simulink library "SG_library"  (R2020a)
settings: Solver=VariableStepAuto  StartTime=0.0  StopTime=10.0  RelTol=1e-3
undefined symbols (not defined in the file): a, b, c, IO334, IO397
libraries: speedgoatlib_hdlCoder_IO3xx x54, $bdroot x8, hdlsllib x7, simulink x1, simulink_extras x1
(part 1 of 2)
settings Model: Creator=mavolery  LastModifiedBy=padlewsk
settings SFSimCC: CustomCodeUndefinedFunction=UseInterfaceOnly

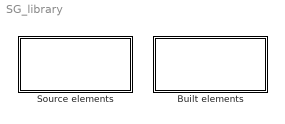
== system SG_library ==
  Built elements : Subsystem
  Source elements : Subsystem

== system SG_library/Built elements ==
  IO334_IO : Subsystem  mask(IO334 IO){}
      mask help: Links the four first physical analog inputs/outputs to the CPU part of the speedgoat.
  IO334_SOS : Subsystem  mask(IO334 M){}
      mask help: Implements a discrete fixed-point filter by second order sections cascade. SOS matrices are given by tf2sos or zp2sos.
  IO397_IO : Subsystem  mask(IO334 IO){}
      mask help: Links the four first physical analog inputs/outputs to the CPU part of the speedgoat.
  IO397_SOS : Subsystem  mask(IO334 IO){}
      mask help: Links the four first physical analog inputs/outputs to the CPU part of the speedgoat.

== system SG_library/Source elements ==
  ADC trigger : Subsystem  mask(AI trigger){}
      mask help: Creates a boolean pulse every given cylces. It can be use for ADC acquisition
  ADC trigger held : Subsystem  mask(AI trigger held){nHeld=2}
      mask prompts: nHeld "Cycles held"
      mask help: Creates a boolean pulse on 'trig' every given cylces. It can be use for ADC acquisition. On 'trig_held' the signal is held to have a for a given number of cycles.
  Discrete SOS section FXP : Subsystem  mask(Discrete fixed-point SOS section){idx=1}
      mask prompts: idx "Index"
      mask help:
      | This is a fixed-point implementation of a biquad filter. Specify the sos [N/2, 6] matrix e.g. given by tf2sos or zpk2sos functions. The first denominator coefficient must always be equal to 1. Index (1 - N/2) parameter specifies which section of the filter is implemented.
      |
      | This is the same implementation as in LabView VI "Discrete Transfer Function Direct.vi" or order 2. It has same fixed-point implementation too.
  Discrete SOS FXP : Subsystem  mask(Discrete fixed-point second order sections filter){sigDataType=fixdt(1,32,16), coefDataType=fixdt(1,32,20)}
      mask prompts: sigDataType "Signal data type"; coefDataType "Coef. data type"
      mask help: This is a SOS implemetation of order 8 (4 sections). Specify the sos [n/2, 6] matrix e.g. given by tf2sos function. The first denominator coefficient must always be equal to 1.
      mask DialogControl Container2 Prompt: Parameters
  Get ADC ticks : Subsystem  mask(Get ADC ticks){}
      mask help: Returns the nuber of FPGA cycles between two ADC acquisitions, given the FPGA clock freuency, the FPGA oversampling factor and the desired acquisition rate.
  Random source : Subsystem  mask(Random source){mean=0, stdev=1, seed=0, SampleTime=0.0001}
      mask prompts: stdev "Standard deviation"; SampleTime "Sample time"
      mask help: Creates some random signal, limited in frequency at Fs/4
  Resettable unit delay : Subsystem  mask(Resettable unit delay){}
      mask Display: dpoly([0 1],[1 0],'z');
  Triggered Pulse : Subsystem  mask(Triggered Pulse){}
      mask help: Generates a single pulse of N samples length

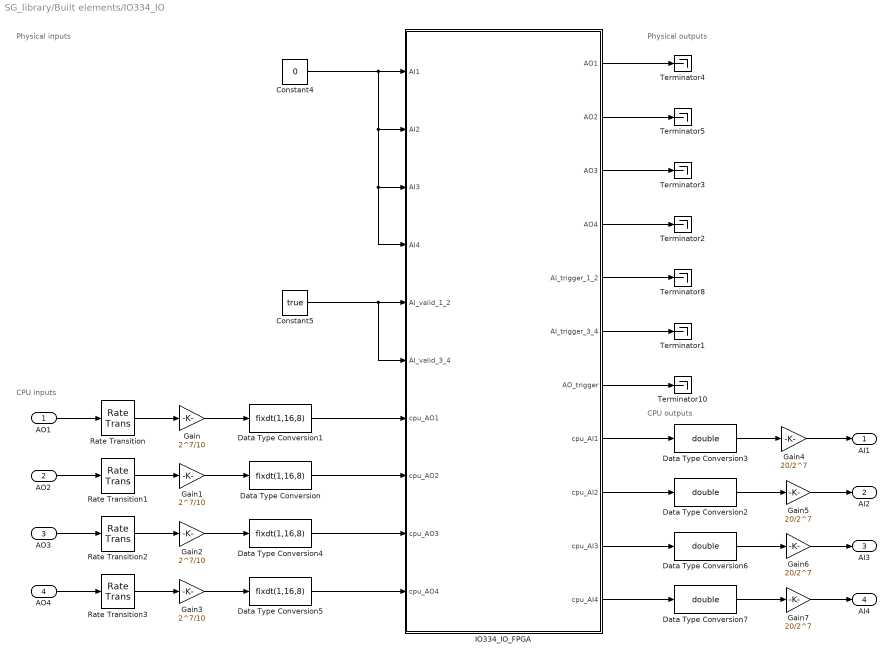
== system SG_library/Built elements/IO334_IO ==
  note: CPU outputs
  note: Physical outputs
  note: Physical inputs
  note: CPU inputs
  AO1 : Inport
  AO2 : Inport  Port=2
  AO3 : Inport  Port=3
  AO4 : Inport  Port=4
  Constant4 : Constant  Value=0  OutDataTypeStr=fixdt(1,16,8)  SampleTime=-1
  Constant5 : Constant  Value=true  SampleTime=-1
  Data Type Conversion{,1,4..5} (4 alike) : DataTypeConversion  OutDataTypeStr=fixdt(1,16,8)
  Data Type Conversion{2..3,6..7} (4 alike) : DataTypeConversion  OutDataTypeStr=double
  Gain{,1..3} (4 alike) : Gain  Gain=2^7/10
  Gain{4..7} (4 alike) : Gain  Gain=20/2^7
  IO334_IO_FPGA : Subsystem  mask(Speedgoat IO334-325k Interface Block){module_id=1, slot=-1, ts=-1, OutputRange=Auto (same as ADC), FpgaFreq=100}
      mask prompts: module_id "FPGA Module Identifier:"; slot "PCI slot (-1: autosearch):"; ts "Sample time:"; OutputRange "DAC Voltage Range:"; FpgaFreq "FPGA Frequency [MHz]"
      mask help: Simulink Real-Time Interface Block for Speedgoat IO334-325k.
      mask init:
      | mfpgaparameters;
      mask Help: eval('speedgoatdoc_hdlc')
      mask TypeOptions OutputRange: IO334 DAC Setup/OutputRange
      mask DialogControl AnalogOutput Prompt: Analog Output
      mask Display:
      | SetupBlkPath = find_system(gcb, 'LookUnderMasks', 'all', 'FollowLinks', 'on', 'regexp', 'on', 'Name', 'IO3(\d|x){2}\s+Setup' );
      | SetupBlkPath = SetupBlkPath{1};
      | TS = get_param(SetupBlkPath,'timestamp_mcs');
      | disp(sprintf('Speedgoat IO334-325k\nFPGA I/O Module\n\nTimestamp\n%s\n\nReference Design\nVersion 1.2\n\nMatlab R2020a\n\nPCIe Link Width: X4\nRear Plugin: None\nAurora Mode: None\nAurora Byteswap: true\n', TS))
  Rate Transition{,1..3} (4 alike) : RateTransition
  Terminator{1..5,8,10} (7 alike) : Terminator
  AI1 : Outport  VectorParamsAs1DForOutWhenUnconnected=off
  AI2 : Outport  Port=2  VectorParamsAs1DForOutWhenUnconnected=off
  AI3 : Outport  Port=3  VectorParamsAs1DForOutWhenUnconnected=off
  AI4 : Outport  Port=4  VectorParamsAs1DForOutWhenUnconnected=off
  wires:
  AO1/1 -> Rate Transition/1
  AO2/1 -> Rate Transition1/1
  Rate Transition/1 -> Gain/1
  Rate Transition1/1 -> Gain1/1
  Data Type Conversion3/1 -> Gain4/1
  Data Type Conversion2/1 -> Gain5/1
  Rate Transition2/1 -> Gain2/1
  AO3/1 -> Rate Transition2/1
  Rate Transition3/1 -> Gain3/1
  AO4/1 -> Rate Transition3/1
  Data Type Conversion5/1 -> IO334_IO_FPGA/10(cpu_AO4)
  Data Type Conversion/1 -> IO334_IO_FPGA/8(cpu_AO2)
  Data Type Conversion4/1 -> IO334_IO_FPGA/9(cpu_AO3)
  Data Type Conversion1/1 -> IO334_IO_FPGA/7(cpu_AO1)
  Data Type Conversion6/1 -> Gain6/1
  Data Type Conversion7/1 -> Gain7/1
  IO334_IO_FPGA/1(AO1) -> Terminator4/1
  IO334_IO_FPGA/8(cpu_AI1) -> Data Type Conversion3/1
  IO334_IO_FPGA/9(cpu_AI2) -> Data Type Conversion2/1
  IO334_IO_FPGA/10(cpu_AI3) -> Data Type Conversion6/1
  IO334_IO_FPGA/11(cpu_AI4) -> Data Type Conversion7/1
  IO334_IO_FPGA/7(AO_trigger) -> Terminator10/1
  IO334_IO_FPGA/6(AI_trigger_3_4) -> Terminator1/1
  IO334_IO_FPGA/5(AI_trigger_1_2) -> Terminator8/1
  IO334_IO_FPGA/4(AO4) -> Terminator2/1
  IO334_IO_FPGA/3(AO3) -> Terminator3/1
  IO334_IO_FPGA/2(AO2) -> Terminator5/1
  Gain/1 -> Data Type Conversion1/1
  Gain1/1 -> Data Type Conversion/1
  Gain2/1 -> Data Type Conversion4/1
  Gain3/1 -> Data Type Conversion5/1
  Gain4/1 -> AI1/1
  Gain5/1 -> AI2/1
  Gain6/1 -> AI3/1
  Gain7/1 -> AI4/1
  Constant5/1 -> IO334_IO_FPGA/6(AI_valid_3_4), IO334_IO_FPGA/5(AI_valid_1_2)
  Constant4/1 -> IO334_IO_FPGA/2(AI2), IO334_IO_FPGA/3(AI3), IO334_IO_FPGA/4(AI4), IO334_IO_FPGA/1(AI1)

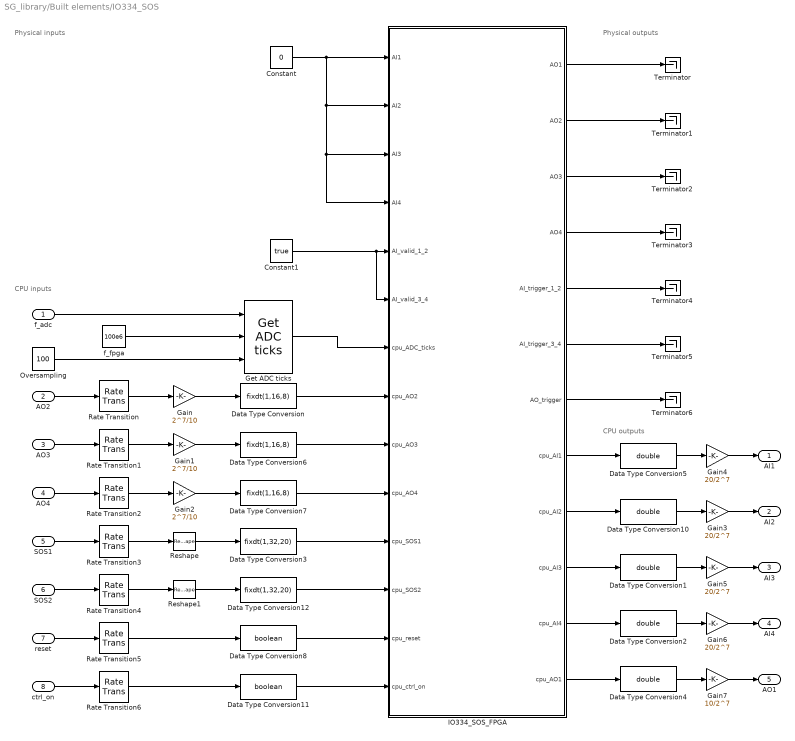
== system SG_library/Built elements/IO334_SOS ==
  note: Physical inputs
  note: CPU inputs
  note: CPU outputs
  note: Physical outputs
  f_adc : Inport
  AO2 : Inport  Port=2
  AO3 : Inport  Port=3
  AO4 : Inport  Port=4
  SOS1 : Inport  Port=5
  SOS2 : Inport  Port=6
  reset : Inport  Port=7
  ctrl_on : Inport  Port=8
  Constant : Constant  Value=0  OutDataTypeStr=fixdt(1,16,8)  SampleTime=-1
  Constant1 : Constant  Value=true  SampleTime=-1
  Data Type Conversion : DataTypeConversion  OutDataTypeStr=fixdt(1,16,8)
  Data Type Conversion{1..2,4..5,10} (5 alike) : DataTypeConversion  OutDataTypeStr=double
  Data Type Conversion11 : DataTypeConversion  OutDataTypeStr=boolean
  Data Type Conversion12 : DataTypeConversion  OutDataTypeStr=fixdt(1,32,20)
  Data Type Conversion3 : DataTypeConversion  OutDataTypeStr=fixdt(1,32,20)
  Data Type Conversion6 : DataTypeConversion  OutDataTypeStr=fixdt(1,16,8)
  Data Type Conversion7 : DataTypeConversion  OutDataTypeStr=fixdt(1,16,8)
  Data Type Conversion8 : DataTypeConversion  OutDataTypeStr=boolean
  Gain : Gain  Gain=2^7/10
  Gain1 : Gain  Gain=2^7/10
  Gain2 : Gain  Gain=2^7/10
  Gain{3..6} (4 alike) : Gain  Gain=20/2^7
  Gain7 : Gain  Gain=10/2^7
  Get ADC ticks : $bdroot/Source elements/Get ADC ticks
  IO334_SOS_FPGA : Subsystem  mask(Speedgoat IO334-325k Interface Block){module_id=1, slot=-1, ts=-1, OutputRange=Auto (same as ADC), FpgaFreq=100}
      mask prompts: module_id "FPGA Module Identifier:"; slot "PCI slot (-1: autosearch):"; ts "Sample time:"; OutputRange "DAC Voltage Range:"; FpgaFreq "FPGA Frequency [MHz]"
      mask help: Simulink Real-Time Interface Block for Speedgoat IO334-325k.
      mask init:
      | mfpgaparameters;
      mask Help: eval('speedgoatdoc_hdlc')
      mask TypeOptions OutputRange: IO334 DAC Setup/OutputRange
      mask DialogControl AnalogOutput Prompt: Analog Output
      mask Display:
      | SetupBlkPath = find_system(gcb, 'LookUnderMasks', 'all', 'FollowLinks', 'on', 'regexp', 'on', 'Name', 'IO3(\d|x){2}\s+Setup' );
      | SetupBlkPath = SetupBlkPath{1};
      | TS = get_param(SetupBlkPath,'timestamp_mcs');
      | disp(sprintf('Speedgoat IO334-325k\nFPGA I/O Module\n\nTimestamp\n%s\n\nReference Design\nVersion 1.2\n\nMatlab R2020a\n\nPCIe Link Width: X4\nRear Plugin: None\nAurora Mode: None\nAurora Byteswap: true\n', TS))
  Oversampling : Constant  Value=100  SampleTime=-1
  Rate Transition{,1..6} (7 alike) : RateTransition
  Reshape : Reshape
  Reshape1 : Reshape
  Terminator{,1..6} (7 alike) : Terminator
  f_fpga : Constant  Value=100e6  SampleTime=-1
  AI1 : Outport  VectorParamsAs1DForOutWhenUnconnected=off
  AI2 : Outport  Port=2  VectorParamsAs1DForOutWhenUnconnected=off
  AI3 : Outport  Port=3  VectorParamsAs1DForOutWhenUnconnected=off
  AI4 : Outport  Port=4  VectorParamsAs1DForOutWhenUnconnected=off
  AO1 : Outport  Port=5  VectorParamsAs1DForOutWhenUnconnected=off
  wires:
  Data Type Conversion10/1 -> Gain3/1
  Data Type Conversion5/1 -> Gain4/1
  Data Type Conversion1/1 -> Gain5/1
  Data Type Conversion2/1 -> Gain6/1
  IO334_SOS_FPGA/1(AO1) -> Terminator/1
  IO334_SOS_FPGA/2(AO2) -> Terminator1/1
  IO334_SOS_FPGA/3(AO3) -> Terminator2/1
  IO334_SOS_FPGA/4(AO4) -> Terminator3/1
  IO334_SOS_FPGA/5(AI_trigger_1_2) -> Terminator4/1
  IO334_SOS_FPGA/6(AI_trigger_3_4) -> Terminator5/1
  IO334_SOS_FPGA/7(AO_trigger) -> Terminator6/1
  IO334_SOS_FPGA/8(cpu_AI1) -> Data Type Conversion5/1
  IO334_SOS_FPGA/9(cpu_AI2) -> Data Type Conversion10/1
  IO334_SOS_FPGA/10(cpu_AI3) -> Data Type Conversion1/1
  IO334_SOS_FPGA/11(cpu_AI4) -> Data Type Conversion2/1
  Rate Transition3/1 -> Reshape/1
  Rate Transition/1 -> Gain/1
  Rate Transition1/1 -> Gain1/1
  Rate Transition2/1 -> Gain2/1
  AO2/1 -> Rate Transition/1
  AO3/1 -> Rate Transition1/1
  AO4/1 -> Rate Transition2/1
  Rate Transition5/1 -> Data Type Conversion8/1
  reset/1 -> Rate Transition5/1
  Rate Transition6/1 -> Data Type Conversion11/1
  ctrl_on/1 -> Rate Transition6/1
  Data Type Conversion/1 -> IO334_SOS_FPGA/8(cpu_AO2)
  Data Type Conversion6/1 -> IO334_SOS_FPGA/9(cpu_AO3)
  Data Type Conversion7/1 -> IO334_SOS_FPGA/10(cpu_AO4)
  Data Type Conversion11/1 -> IO334_SOS_FPGA/14(cpu_ctrl_on)
  Data Type Conversion8/1 -> IO334_SOS_FPGA/13(cpu_reset)
  Constant1/1 -> IO334_SOS_FPGA/5(AI_valid_1_2), IO334_SOS_FPGA/6(AI_valid_3_4)
  Constant/1 -> IO334_SOS_FPGA/1(AI1), IO334_SOS_FPGA/2(AI2), IO334_SOS_FPGA/3(AI3), IO334_SOS_FPGA/4(AI4)
  SOS1/1 -> Rate Transition3/1
  Data Type Conversion3/1 -> IO334_SOS_FPGA/11(cpu_SOS1)
  f_adc/1 -> Get ADC ticks/1
  Oversampling/1 -> Get ADC ticks/3
  f_fpga/1 -> Get ADC ticks/2
  Data Type Conversion4/1 -> Gain7/1
  IO334_SOS_FPGA/12(cpu_AO1) -> Data Type Conversion4/1
  Rate Transition4/1 -> Reshape1/1
  SOS2/1 -> Rate Transition4/1
  Data Type Conversion12/1 -> IO334_SOS_FPGA/12(cpu_SOS2)
  Gain/1 -> Data Type Conversion/1
  Gain1/1 -> Data Type Conversion6/1
  Gain2/1 -> Data Type Conversion7/1
  Reshape/1 -> Data Type Conversion3/1
  Reshape1/1 -> Data Type Conversion12/1
  Get ADC ticks/1 -> IO334_SOS_FPGA/7(cpu_ADC_ticks)
  Gain4/1 -> AI1/1
  Gain3/1 -> AI2/1
  Gain5/1 -> AI3/1
  Gain6/1 -> AI4/1
  Gain7/1 -> AO1/1

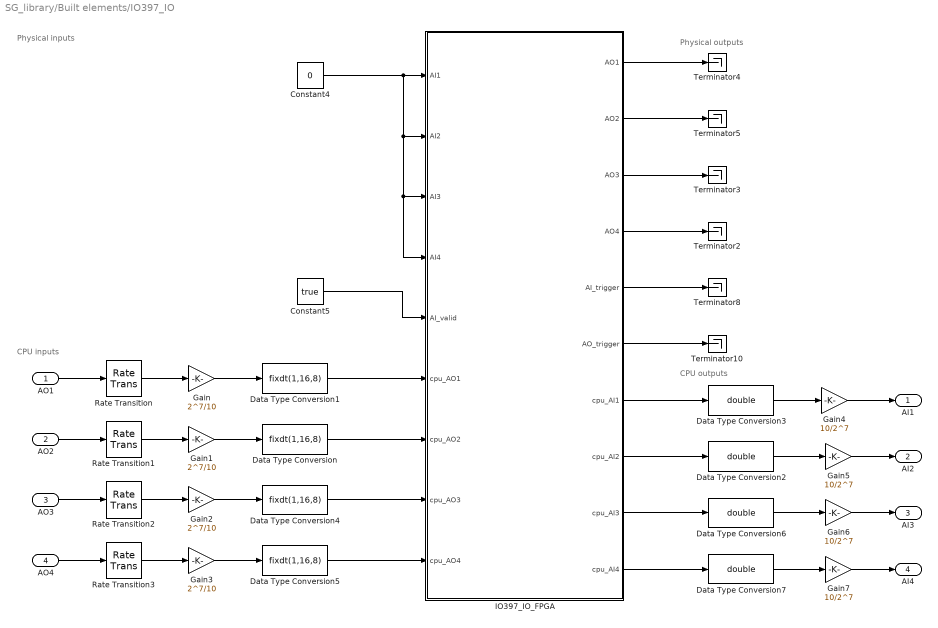
== system SG_library/Built elements/IO397_IO ==
  note: CPU outputs
  note: Physical outputs
  note: Physical inputs
  note: CPU inputs
  AO1 : Inport
  AO2 : Inport  Port=2
  AO3 : Inport  Port=3
  AO4 : Inport  Port=4
  Constant4 : Constant  Value=0  OutDataTypeStr=fixdt(1,16,8)  SampleTime=-1
  Constant5 : Constant  Value=true  SampleTime=-1
  Data Type Conversion{,1,4..5} (4 alike) : DataTypeConversion  OutDataTypeStr=fixdt(1,16,8)  SaturateOnIntegerOverflow=on
  Data Type Conversion{2..3,6..7} (4 alike) : DataTypeConversion  OutDataTypeStr=double
  Gain{,1..3} (4 alike) : Gain  Gain=2^7/10
  Gain{4..7} (4 alike) : Gain  Gain=10/2^7
  IO397_IO_FPGA : Subsystem  mask(Speedgoat IO397-50k Interface Block){module_id=1, slot=-1, ts=-1, range1=+-10 V, range2=+-10 V, range3=+-10 V, range4=+-10 V, span=+-10 V, FpgaFreq=100}
      mask prompts: module_id "FPGA Module Identifier:"; slot "PCI slot (-1: autosearch):"; ts "Sample time:"; range1 "Range ADC Channel 1"; range2 "Range ADC Channel 2"; range3 "Range ADC Channel 3"; range4 "Range ADC Channel 4"; span "DAC Voltage Span:"; FpgaFreq "FPGA Frequency [MHz]"
      mask help: Simulink Real-Time Interface Block for Speedgoat IO397-50k.
      mask init:
      | mfpgaparameters;
      mask Help: eval('speedgoatdoc_hdlc')
      mask TypeOptions range1: IO397 ADC Setup/range1
      mask TypeOptions range2: IO397 ADC Setup/range2
      mask TypeOptions range3: IO397 ADC Setup/range3
      mask TypeOptions range4: IO397 ADC Setup/range4
      mask TypeOptions span: IO397 DAC Setup/span
      mask DialogControl AnalogInput Prompt: Analog Input
      mask DialogControl AnalogOutput Prompt: Analog Output
      mask Display:
      | SetupBlkPath = find_system(gcb, 'LookUnderMasks', 'all', 'FollowLinks', 'on', 'regexp', 'on', 'Name', 'IO3(\d|x){2}\s+Setup' );
      | SetupBlkPath = SetupBlkPath{1};
      | TS = get_param(SetupBlkPath,'timestamp_mcs');
      | disp(sprintf('Speedgoat IO397-50k\nFPGA I/O Module\n\nTimestamp\n%s\n\nReference Design\nVersion 1.2\n\nMatlab R2020a\n\nPCIe Link Width: X1\n', TS))
  Rate Transition{,1..3} (4 alike) : RateTransition
  Terminator{2..5,8,10} (6 alike) : Terminator
  AI1 : Outport  VectorParamsAs1DForOutWhenUnconnected=off
  AI2 : Outport  Port=2  VectorParamsAs1DForOutWhenUnconnected=off
  AI3 : Outport  Port=3  VectorParamsAs1DForOutWhenUnconnected=off
  AI4 : Outport  Port=4  VectorParamsAs1DForOutWhenUnconnected=off
  wires:
  AO1/1 -> Rate Transition/1
  AO2/1 -> Rate Transition1/1
  Rate Transition/1 -> Gain/1
  Rate Transition1/1 -> Gain1/1
  Data Type Conversion3/1 -> Gain4/1
  Data Type Conversion2/1 -> Gain5/1
  Rate Transition2/1 -> Gain2/1
  AO3/1 -> Rate Transition2/1
  Rate Transition3/1 -> Gain3/1
  AO4/1 -> Rate Transition3/1
  Data Type Conversion5/1 -> IO397_IO_FPGA/9(cpu_AO4)
  Data Type Conversion/1 -> IO397_IO_FPGA/7(cpu_AO2)
  Data Type Conversion4/1 -> IO397_IO_FPGA/8(cpu_AO3)
  Data Type Conversion1/1 -> IO397_IO_FPGA/6(cpu_AO1)
  Data Type Conversion6/1 -> Gain6/1
  Data Type Conversion7/1 -> Gain7/1
  IO397_IO_FPGA/1(AO1) -> Terminator4/1
  IO397_IO_FPGA/7(cpu_AI1) -> Data Type Conversion3/1
  IO397_IO_FPGA/8(cpu_AI2) -> Data Type Conversion2/1
  IO397_IO_FPGA/9(cpu_AI3) -> Data Type Conversion6/1
  IO397_IO_FPGA/10(cpu_AI4) -> Data Type Conversion7/1
  IO397_IO_FPGA/6(AO_trigger) -> Terminator10/1
  IO397_IO_FPGA/5(AI_trigger) -> Terminator8/1
  IO397_IO_FPGA/4(AO4) -> Terminator2/1
  IO397_IO_FPGA/3(AO3) -> Terminator3/1
  IO397_IO_FPGA/2(AO2) -> Terminator5/1
  Gain/1 -> Data Type Conversion1/1
  Gain1/1 -> Data Type Conversion/1
  Gain2/1 -> Data Type Conversion4/1
  Gain3/1 -> Data Type Conversion5/1
  Gain4/1 -> AI1/1
  Gain5/1 -> AI2/1
  Gain6/1 -> AI3/1
  Gain7/1 -> AI4/1
  Constant5/1 -> IO397_IO_FPGA/5(AI_valid)
  Constant4/1 -> IO397_IO_FPGA/2(AI2), IO397_IO_FPGA/3(AI3), IO397_IO_FPGA/4(AI4), IO397_IO_FPGA/1(AI1)

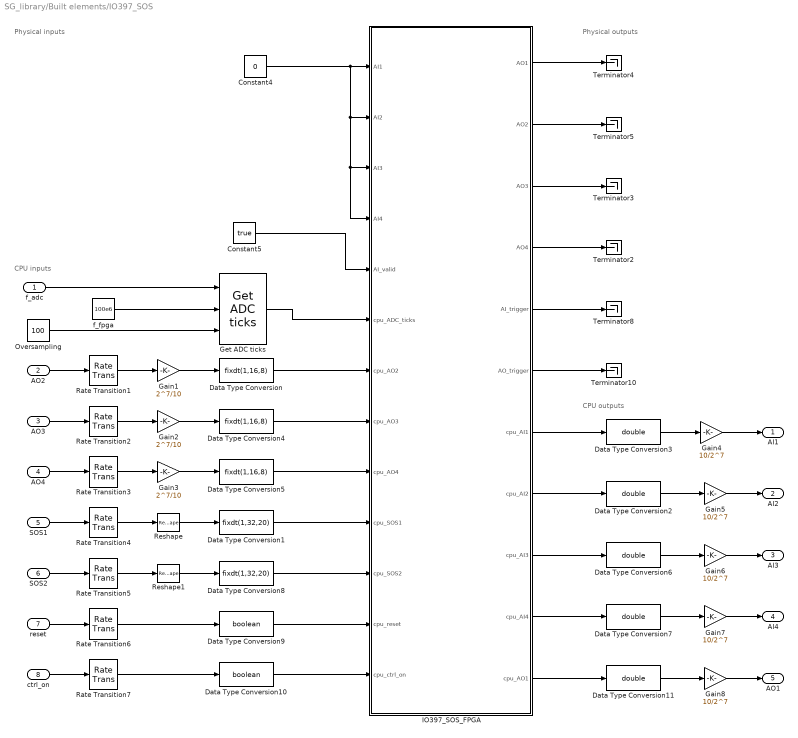
== system SG_library/Built elements/IO397_SOS ==
  note: CPU outputs
  note: Physical outputs
  note: Physical inputs
  note: CPU inputs
  f_adc : Inport
  AO2 : Inport  Port=2
  AO3 : Inport  Port=3
  AO4 : Inport  Port=4
  SOS1 : Inport  Port=5
  SOS2 : Inport  Port=6
  reset : Inport  Port=7
  ctrl_on : Inport  Port=8
  Constant4 : Constant  Value=0  OutDataTypeStr=fixdt(1,16,8)  SampleTime=-1
  Constant5 : Constant  Value=true  SampleTime=-1
  Data Type Conversion : DataTypeConversion  OutDataTypeStr=fixdt(1,16,8)  SaturateOnIntegerOverflow=on
  Data Type Conversion1 : DataTypeConversion  OutDataTypeStr=fixdt(1,32,20)  SaturateOnIntegerOverflow=on
  Data Type Conversion10 : DataTypeConversion  OutDataTypeStr=boolean
  Data Type Conversion{2..3,6..7,11} (5 alike) : DataTypeConversion  OutDataTypeStr=double
  Data Type Conversion4 : DataTypeConversion  OutDataTypeStr=fixdt(1,16,8)  SaturateOnIntegerOverflow=on
  Data Type Conversion5 : DataTypeConversion  OutDataTypeStr=fixdt(1,16,8)  SaturateOnIntegerOverflow=on
  Data Type Conversion8 : DataTypeConversion  OutDataTypeStr=fixdt(1,32,20)  SaturateOnIntegerOverflow=on
  Data Type Conversion9 : DataTypeConversion  OutDataTypeStr=boolean
  Gain1 : Gain  Gain=2^7/10
  Gain2 : Gain  Gain=2^7/10
  Gain3 : Gain  Gain=2^7/10
  Gain{4..8} (5 alike) : Gain  Gain=10/2^7
  Get ADC ticks : $bdroot/Source elements/Get ADC ticks
  IO397_SOS_FPGA : Subsystem  mask(Speedgoat IO397-50k Interface Block){module_id=1, slot=-1, ts=-1, range1=+-10 V, range2=+-10 V, range3=+-10 V, range4=+-10 V, span=+-10 V, FpgaFreq=100}
      mask prompts: module_id "FPGA Module Identifier:"; slot "PCI slot (-1: autosearch):"; ts "Sample time:"; range1 "Range ADC Channel 1"; range2 "Range ADC Channel 2"; range3 "Range ADC Channel 3"; range4 "Range ADC Channel 4"; span "DAC Voltage Span:"; FpgaFreq "FPGA Frequency [MHz]"
      mask help: Simulink Real-Time Interface Block for Speedgoat IO397-50k.
      mask init:
      | mfpgaparameters;
      mask Help: eval('speedgoatdoc_hdlc')
      mask TypeOptions range1: IO397 ADC Setup/range1
      mask TypeOptions range2: IO397 ADC Setup/range2
      mask TypeOptions range3: IO397 ADC Setup/range3
      mask TypeOptions range4: IO397 ADC Setup/range4
      mask TypeOptions span: IO397 DAC Setup/span
      mask DialogControl AnalogInput Prompt: Analog Input
      mask DialogControl AnalogOutput Prompt: Analog Output
      mask Display:
      | SetupBlkPath = find_system(gcb, 'LookUnderMasks', 'all', 'FollowLinks', 'on', 'regexp', 'on', 'Name', 'IO3(\d|x){2}\s+Setup' );
      | SetupBlkPath = SetupBlkPath{1};
      | TS = get_param(SetupBlkPath,'timestamp_mcs');
      | disp(sprintf('Speedgoat IO397-50k\nFPGA I/O Module\n\nTimestamp\n%s\n\nReference Design\nVersion 1.2\n\nMatlab R2020a\n\nPCIe Link Width: X1\n', TS))
  Oversampling : Constant  Value=100
  Rate Transition{1..7} (7 alike) : RateTransition
  Reshape : Reshape
  Reshape1 : Reshape
  Terminator{2..5,8,10} (6 alike) : Terminator
  f_fpga : Constant  Value=100e6
  AI1 : Outport  VectorParamsAs1DForOutWhenUnconnected=off
  AI2 : Outport  Port=2  VectorParamsAs1DForOutWhenUnconnected=off
  AI3 : Outport  Port=3  VectorParamsAs1DForOutWhenUnconnected=off
  AI4 : Outport  Port=4  VectorParamsAs1DForOutWhenUnconnected=off
  AO1 : Outport  Port=5  VectorParamsAs1DForOutWhenUnconnected=off
  wires:
  AO2/1 -> Rate Transition1/1
  Rate Transition1/1 -> Gain1/1
  Data Type Conversion3/1 -> Gain4/1
  Data Type Conversion2/1 -> Gain5/1
  Rate Transition2/1 -> Gain2/1
  AO3/1 -> Rate Transition2/1
  Rate Transition3/1 -> Gain3/1
  AO4/1 -> Rate Transition3/1
  Data Type Conversion5/1 -> IO397_SOS_FPGA/9(cpu_AO4)
  Data Type Conversion/1 -> IO397_SOS_FPGA/7(cpu_AO2)
  Data Type Conversion4/1 -> IO397_SOS_FPGA/8(cpu_AO3)
  Data Type Conversion6/1 -> Gain6/1
  Data Type Conversion7/1 -> Gain7/1
  IO397_SOS_FPGA/1(AO1) -> Terminator4/1
  IO397_SOS_FPGA/7(cpu_AI1) -> Data Type Conversion3/1
  IO397_SOS_FPGA/8(cpu_AI2) -> Data Type Conversion2/1
  IO397_SOS_FPGA/9(cpu_AI3) -> Data Type Conversion6/1
  IO397_SOS_FPGA/10(cpu_AI4) -> Data Type Conversion7/1
  IO397_SOS_FPGA/6(AO_trigger) -> Terminator10/1
  IO397_SOS_FPGA/5(AI_trigger) -> Terminator8/1
  IO397_SOS_FPGA/4(AO4) -> Terminator2/1
  IO397_SOS_FPGA/3(AO3) -> Terminator3/1
  IO397_SOS_FPGA/2(AO2) -> Terminator5/1
  Gain1/1 -> Data Type Conversion/1
  Gain2/1 -> Data Type Conversion4/1
  Gain3/1 -> Data Type Conversion5/1
  Gain4/1 -> AI1/1
  Gain5/1 -> AI2/1
  Gain6/1 -> AI3/1
  Gain7/1 -> AI4/1
  Constant5/1 -> IO397_SOS_FPGA/5(AI_valid)
  Constant4/1 -> IO397_SOS_FPGA/3(AI3), IO397_SOS_FPGA/4(AI4), IO397_SOS_FPGA/2(AI2), IO397_SOS_FPGA/1(AI1)
  ctrl_on/1 -> Rate Transition7/1
  reset/1 -> Rate Transition6/1
  SOS2/1 -> Rate Transition5/1
  SOS1/1 -> Rate Transition4/1
  f_adc/1 -> Get ADC ticks/1
  f_fpga/1 -> Get ADC ticks/2
  Oversampling/1 -> Get ADC ticks/3
  Rate Transition4/1 -> Reshape/1
  Rate Transition5/1 -> Reshape1/1
  Reshape1/1 -> Data Type Conversion8/1
  Reshape/1 -> Data Type Conversion1/1
  Rate Transition6/1 -> Data Type Conversion9/1
  Rate Transition7/1 -> Data Type Conversion10/1
  Data Type Conversion9/1 -> IO397_SOS_FPGA/12(cpu_reset)
  Data Type Conversion10/1 -> IO397_SOS_FPGA/13(cpu_ctrl_on)
  Data Type Conversion8/1 -> IO397_SOS_FPGA/11(cpu_SOS2)
  Data Type Conversion1/1 -> IO397_SOS_FPGA/10(cpu_SOS1)
  Get ADC ticks/1 -> IO397_SOS_FPGA/6(cpu_ADC_ticks)
  Data Type Conversion11/1 -> Gain8/1
  Gain8/1 -> AO1/1
  IO397_SOS_FPGA/11(cpu_AO1) -> Data Type Conversion11/1

== system SG_library/Source elements/ADC trigger ==
  ticks : Inport
  HDL Counter3 : hdlsllib/Sources/HDL Counter  CountType=Free running  CountInit=uint32(0)  CountStep=uint32(1)  CountMax=25  CountFromType=Initial value  CountFrom=uint32(0)  CountResetPort=on  CountLoadPort=off  CountEnbPort=off  CountDirPort=off  CountDataType=Unsigned  CountWordLen=32  CountFracLen=0  CountSampTime=1
  Relational Operator1 : RelationalOperator  Operator=<=  OutDataTypeStr=boolean  RndMeth=Simplest
  trig : Outport  VectorParamsAs1DForOutWhenUnconnected=off
  wires:
  HDL Counter3/1 -> Relational Operator1/2
  ticks/1 -> Relational Operator1/1
  Relational Operator1/1 -> HDL Counter3/1, trig/1

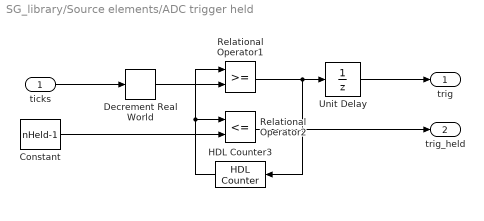
== system SG_library/Source elements/ADC trigger held ==
  ticks : Inport
  Constant : Constant  Value=nHeld-1  OutDataTypeStr=uint32  SampleTime=-1
  Decrement Real World : simulink/Additional Math & Discrete/Additional Math: Increment - Decrement/Decrement Real World
      settings: SourceProductBaseCode=SL
  HDL Counter3 : hdlsllib/Sources/HDL Counter  CountType=Free running  CountInit=uint32(0)  CountStep=uint32(1)  CountMax=25  CountFromType=Initial value  CountFrom=uint32(0)  CountResetPort=on  CountLoadPort=off  CountEnbPort=off  CountDirPort=off  CountDataType=Unsigned  CountWordLen=32  CountFracLen=0  CountSampTime=1
  Relational Operator1 : RelationalOperator  OutDataTypeStr=boolean  RndMeth=Simplest
  Relational Operator2 : RelationalOperator  Operator=<=  OutDataTypeStr=boolean  RndMeth=Simplest
  Unit Delay : UnitDelay  SampleTime=-1  HasFrameUpgradeWarning=on
  trig : Outport  VectorParamsAs1DForOutWhenUnconnected=off
  trig_held : Outport  Port=2  VectorParamsAs1DForOutWhenUnconnected=off
  wires:
  HDL Counter3/1 -> Relational Operator1/1, Relational Operator2/1
  Relational Operator2/1 -> trig_held/1
  Relational Operator1/1 -> Unit Delay/1, HDL Counter3/1
  Unit Delay/1 -> trig/1
  Decrement Real World/1 -> Relational Operator1/2
  ticks/1 -> Decrement Real World/1
  Constant/1 -> Relational Operator2/2

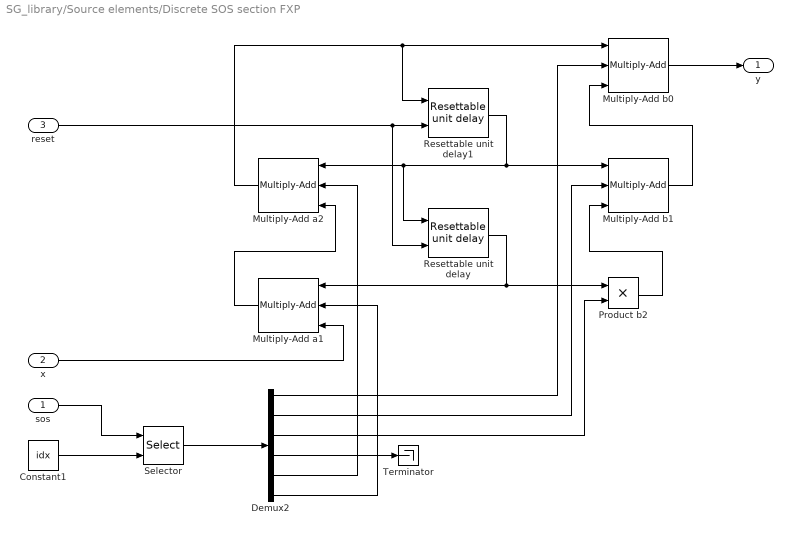
== system SG_library/Source elements/Discrete SOS section FXP ==
  sos : Inport
  x : Inport  Port=2
  reset : Inport  Port=3
  Constant1 : Constant  Value=idx  OutDataTypeStr=uint8  SampleTime=-1
  Demux2 : Demux  Outputs=6
  Multiply-Add a1 : hdlsllib/HDL Operations/Multiply-Add  Function=c-(a.*b)  datatype=Inherit: Same as first input  RndMeth=Simplest  DoSatur=on  FMA=off
      settings: SourceProductBaseCode=SL
  Multiply-Add a2 : hdlsllib/HDL Operations/Multiply-Add  Function=c-(a.*b)  datatype=Inherit: Same as first input  RndMeth=Simplest  DoSatur=on  FMA=off
      settings: SourceProductBaseCode=SL
  Multiply-Add b0 : hdlsllib/HDL Operations/Multiply-Add  Function=c+(a.*b)  datatype=Inherit: Same as first input  RndMeth=Simplest  DoSatur=on  FMA=off
      settings: SourceProductBaseCode=SL
  Multiply-Add b1 : hdlsllib/HDL Operations/Multiply-Add  Function=c+(a.*b)  datatype=Inherit: Same as first input  RndMeth=Simplest  DoSatur=on  FMA=off
      settings: SourceProductBaseCode=SL
  Product b2 : Product  RndMeth=Simplest  SaturateOnIntegerOverflow=on  OutDataTypeStr=Inherit: Same as first input
  Resettable unit delay : $bdroot/Source elements/Resettable unit delay  SystemSampleTime=-1  Latency=0  AutoFrameSizeCalculation=off
  Resettable unit delay1 : $bdroot/Source elements/Resettable unit delay  SystemSampleTime=-1  Latency=0  AutoFrameSizeCalculation=off
  Selector : Selector  NumberOfDimensions=2  InputPortWidth=3  IndexOptions=Index vector (port),Select all  Indices=[1 3],[1, 2, 3, 4, 5]  OutputSizes=1,1
  Terminator : Terminator
  y : Outport  InitialOutput=0  VectorParamsAs1DForOutWhenUnconnected=off
  wires:
  Demux2/3 -> Product b2/2
  Demux2/2 -> Multiply-Add b1/2
  Demux2/1 -> Multiply-Add b0/2
  Demux2/5 -> Multiply-Add a2/2
  Constant1/1 -> Selector/2
  Demux2/4 -> Terminator/1
  Selector/1 -> Demux2/1
  sos/1 -> Selector/1
  Demux2/6 -> Multiply-Add a1/2
  Multiply-Add a2/1 -> Resettable unit delay1/1, Multiply-Add b0/1
  reset/1 -> Resettable unit delay1/2, Resettable unit delay/2
  Resettable unit delay1/1 -> Multiply-Add a2/1, Resettable unit delay/1, Multiply-Add b1/1
  Resettable unit delay/1 -> Multiply-Add a1/1, Product b2/1
  Multiply-Add b0/1 -> y/1
  Product b2/1 -> Multiply-Add b1/3
  Multiply-Add b1/1 -> Multiply-Add b0/3
  Multiply-Add a1/1 -> Multiply-Add a2/3
  x/1 -> Multiply-Add a1/3

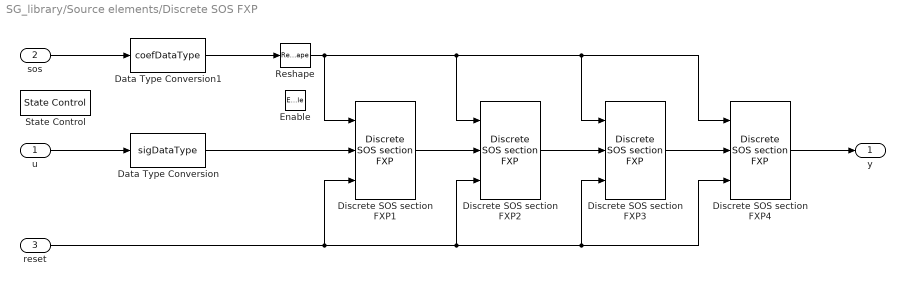
== system SG_library/Source elements/Discrete SOS FXP ==
  u : Inport
  sos : Inport  Port=2
  reset : Inport  Port=3
  Enable : EnablePort
  Data Type Conversion : DataTypeConversion  OutDataTypeStr=sigDataType  RndMeth=Simplest  SaturateOnIntegerOverflow=on
  Data Type Conversion1 : DataTypeConversion  OutDataTypeStr=coefDataType  RndMeth=Simplest  SaturateOnIntegerOverflow=on
  Discrete SOS section FXP1 : $bdroot/Source elements/Discrete SOS section FXP  idx=1
  Discrete SOS section FXP2 : $bdroot/Source elements/Discrete SOS section FXP  idx=2
  Discrete SOS section FXP3 : $bdroot/Source elements/Discrete SOS section FXP  idx=3
  Discrete SOS section FXP4 : $bdroot/Source elements/Discrete SOS section FXP  idx=4
  Reshape : Reshape  OutputDimensionality=Customize  OutputDimensions=[4,6]
  State Control : StateControl  StateControl=Synchronous
  y : Outport  InitialOutput=0  VectorParamsAs1DForOutWhenUnconnected=off
  wires:
  Discrete SOS section FXP2/1 -> Discrete SOS section FXP3/2
  Discrete SOS section FXP3/1 -> Discrete SOS section FXP4/2
  reset/1 -> Discrete SOS section FXP1/3, Discrete SOS section FXP2/3, Discrete SOS section FXP3/3, Discrete SOS section FXP4/3
  Discrete SOS section FXP4/1 -> y/1
  Reshape/1 -> Discrete SOS section FXP1/1, Discrete SOS section FXP2/1, Discrete SOS section FXP3/1, Discrete SOS section FXP4/1
  Discrete SOS section FXP1/1 -> Discrete SOS section FXP2/2
  sos/1 -> Data Type Conversion1/1
  u/1 -> Data Type Conversion/1
  Data Type Conversion1/1 -> Reshape/1
  Data Type Conversion/1 -> Discrete SOS section FXP1/2

== system SG_library/Source elements/Get ADC ticks ==
  f_adc : Inport
  f_fpga : Inport  Port=2
  os : Inport  Port=3
  MATLAB Function : MATLAB Function  TreatAsAtomicUnit=on
  ticks : Outport  VectorParamsAs1DForOutWhenUnconnected=off
  wires:
  MATLAB Function/1(ticks) -> ticks/1
  f_adc/1 -> MATLAB Function/1(f_adc)
  f_fpga/1 -> MATLAB Function/2(f_fpga)
  os/1 -> MATLAB Function/3(os)

== system SG_library/Source elements/Random source ==
  Discrete Filter : DiscreteFilter  Numerator=[0.5 0.5]  Denominator=[1 0.1]  InputProcessing=Columns as channels (frame based)  FilterStructure=Direct form II transposed  a0EqualsOne=on
  Random Number : RandomNumber  Mean=mean  Variance=stdev^2  Seed=seed  SampleTime=SampleTime
  x : Outport  VectorParamsAs1DForOutWhenUnconnected=off
  wires:
  Random Number/1 -> Discrete Filter/1
  Discrete Filter/1 -> x/1

== system SG_library/Source elements/Resettable unit delay ==
  u : Inport
  R : Inport  Port=2
  Constant : Constant  Value=0  OutDataTypeStr=Inherit: Inherit via back propagation  SampleTime=-1
  Switch : Switch  Criteria=u2 > Threshold
  Unit Delay : UnitDelay  SampleTime=-1  HasFrameUpgradeWarning=on
  y : Outport  VectorParamsAs1DForOutWhenUnconnected=off
  wires:
  Switch/1 -> Unit Delay/1
  Constant/1 -> Switch/1
  R/1 -> Switch/2
  u/1 -> Switch/3
  Unit Delay/1 -> y/1

== system SG_library/Source elements/Triggered Pulse ==
  trigger : Inport
  reset : Inport  Port=2
  N : Inport  Port=3
  HDL Counter : hdlsllib/Sources/HDL Counter  CountType=Free running  CountInit=0  CountStep=1  CountMax=25  CountFromType=Initial value  CountFrom=0  CountResetPort=on  CountLoadPort=off  CountEnbPort=on  CountDirPort=off  CountDataType=Unsigned  CountWordLen=32  CountFracLen=0  CountSampTime=1
  OR : Logic  Operator=OR  AllPortsSameDT=off  OutDataTypeStr=boolean
  S-R Flip-Flop : simulink_extras/Flip Flops/S-R Flip-Flop  initial_condition=0
  Terminator : Terminator
  cntr full? : RelationalOperator  OutDataTypeStr=boolean  RndMeth=Simplest
  pulse : Outport  VectorParamsAs1DForOutWhenUnconnected=off
  wires:
  cntr full?/1 -> OR/2
  reset/1 -> OR/1
  OR/1 -> HDL Counter/1, S-R Flip-Flop/2
  S-R Flip-Flop/2 -> Terminator/1
  trigger/1 -> S-R Flip-Flop/1
  N/1 -> cntr full?/2
  S-R Flip-Flop/1 -> HDL Counter/2, pulse/1
  HDL Counter/1 -> cntr full?/1

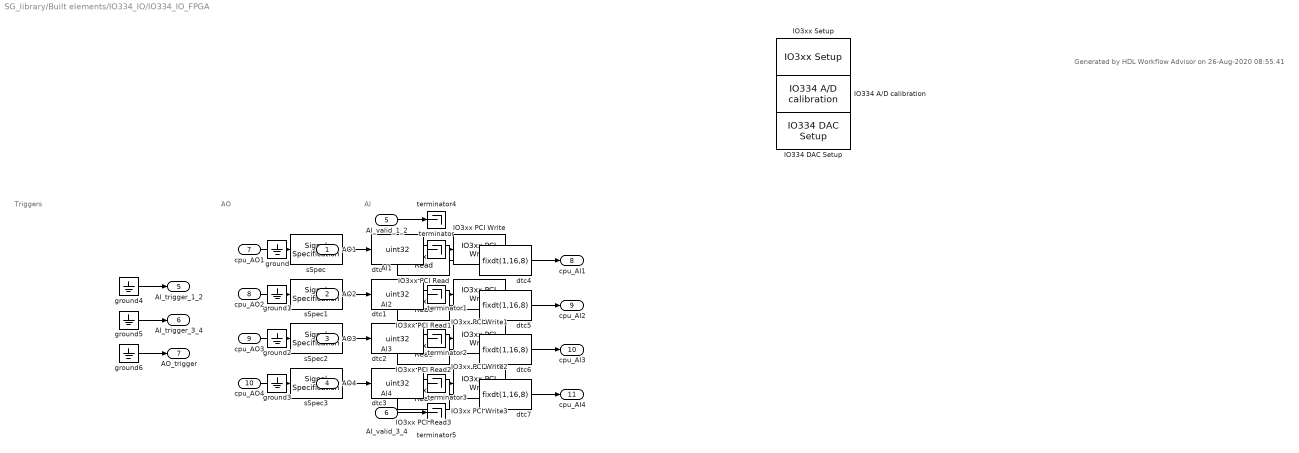
== system SG_library/Built elements/IO334_IO/IO334_IO_FPGA ==
  note: Generated by HDL Workflow Advisor on 26-Aug-2020 08:55:41
  note: Triggers
  note: AI
  note: AO
  AI1 : Inport
  AI2 : Inport  Port=2
  AI3 : Inport  Port=3
  AI4 : Inport  Port=4
  AI_valid_1_2 : Inport  Port=5
  AI_valid_3_4 : Inport  Port=6
  cpu_AO1 : Inport  Port=7
  cpu_AO2 : Inport  Port=8
  cpu_AO3 : Inport  Port=9
  cpu_AO4 : Inport  Port=10
  IO334 A/D calibration : speedgoatlib_hdlCoder_IO3xx/IO334 A//D calibration  module_id=module_id
  IO334 DAC Setup : speedgoatlib_hdlCoder_IO3xx/IO334 DAC Setup  module_id=module_id  OutputRange=Auto (same as ADC)
  IO3xx PCI Read : speedgoatlib_hdlCoder_IO3xx/IO3xx PCI Read  device_id=1  module_id=module_id  board_type=IO334-325k  port_name=cpu_AI1  port_offset=hex2dec('110')  port_type=uint32  port_dim=1  strobe=0  sample_time=ts
  IO3xx PCI Read1 : speedgoatlib_hdlCoder_IO3xx/IO3xx PCI Read  device_id=1  module_id=module_id  board_type=IO334-325k  port_name=cpu_AI2  port_offset=hex2dec('114')  port_type=uint32  port_dim=1  strobe=0  sample_time=ts
  IO3xx PCI Read2 : speedgoatlib_hdlCoder_IO3xx/IO3xx PCI Read  device_id=1  module_id=module_id  board_type=IO334-325k  port_name=cpu_AI3  port_offset=hex2dec('118')  port_type=uint32  port_dim=1  strobe=0  sample_time=ts
  IO3xx PCI Read3 : speedgoatlib_hdlCoder_IO3xx/IO3xx PCI Read  device_id=1  module_id=module_id  board_type=IO334-325k  port_name=cpu_AI4  port_offset=hex2dec('11C')  port_type=uint32  port_dim=1  strobe=0  sample_time=ts
  IO3xx PCI Write : speedgoatlib_hdlCoder_IO3xx/IO3xx PCI Write  device_id=1  module_id=module_id  board_type=IO334-325k  port_name=cpu_AO1  port_offset=hex2dec('100')  port_type=uint32  port_dim=1  strobe=0  sample_time=ts
  IO3xx PCI Write1 : speedgoatlib_hdlCoder_IO3xx/IO3xx PCI Write  device_id=1  module_id=module_id  board_type=IO334-325k  port_name=cpu_AO2  port_offset=hex2dec('104')  port_type=uint32  port_dim=1  strobe=0  sample_time=ts
  IO3xx PCI Write2 : speedgoatlib_hdlCoder_IO3xx/IO3xx PCI Write  device_id=1  module_id=module_id  board_type=IO334-325k  port_name=cpu_AO3  port_offset=hex2dec('108')  port_type=uint32  port_dim=1  strobe=0  sample_time=ts
  IO3xx PCI Write3 : speedgoatlib_hdlCoder_IO3xx/IO3xx PCI Write  device_id=1  module_id=module_id  board_type=IO334-325k  port_name=cpu_AO4  port_offset=hex2dec('10C')  port_type=uint32  port_dim=1  strobe=0  sample_time=ts
  IO3xx Setup : speedgoatlib_hdlCoder_IO3xx/IO3xx Setup  mdl_ss_name=IO334_IO_src/IO334_IO/IO334_IO_FPGA  board_type=IO334-325k  fpga_sync_mode=on  reset_mode=on  device_id=1  module_id=module_id  pci_slot=slot  fpga_mat_file=C:\Speedgoat\Build\IO334_IO\hdlsrc\IO334_IO_src\IO334_IO_FPGA.mat  timestamp_mcs=08/25/20 18:50:46  timestamp=2008251758  tsreg=hex2dec('8')  bsf_file=IO334_IO_FPGA_2008251758.mcs  mcs=0
  dtc{,1..3} (4 alike) : DataTypeConversion  OutDataTypeStr=uint32  ConvertRealWorld=Stored Integer (SI)  RndMeth=Zero
  dtc{4..7} (4 alike) : DataTypeConversion  OutDataTypeStr=fixdt(1,16,8)  ConvertRealWorld=Stored Integer (SI)  RndMeth=Zero
  ground{,1..6} (7 alike) : Ground
  sSpec{,1..3} (4 alike) : SignalSpecification  OutDataTypeStr=fixdt(1,16,8)
  terminator{,1..5} (6 alike) : Terminator
  AO1 : Outport  VectorParamsAs1DForOutWhenUnconnected=off
  AO2 : Outport  Port=2  VectorParamsAs1DForOutWhenUnconnected=off
  AO3 : Outport  Port=3  VectorParamsAs1DForOutWhenUnconnected=off
  AO4 : Outport  Port=4  VectorParamsAs1DForOutWhenUnconnected=off
  AI_trigger_1_2 : Outport  Port=5  VectorParamsAs1DForOutWhenUnconnected=off
  AI_trigger_3_4 : Outport  Port=6  VectorParamsAs1DForOutWhenUnconnected=off
  AO_trigger : Outport  Port=7  VectorParamsAs1DForOutWhenUnconnected=off
  cpu_AI1 : Outport  Port=8  VectorParamsAs1DForOutWhenUnconnected=off
  cpu_AI2 : Outport  Port=9  VectorParamsAs1DForOutWhenUnconnected=off
  cpu_AI3 : Outport  Port=10  VectorParamsAs1DForOutWhenUnconnected=off
  cpu_AI4 : Outport  Port=11  VectorParamsAs1DForOutWhenUnconnected=off
  wires:
  IO3xx PCI Read3/1 -> dtc7/1
  dtc7/1 -> cpu_AI4/1
  IO3xx PCI Read2/1 -> dtc6/1
  dtc6/1 -> cpu_AI3/1
  IO3xx PCI Read1/1 -> dtc5/1
  dtc5/1 -> cpu_AI2/1
  IO3xx PCI Read/1 -> dtc4/1
  dtc4/1 -> cpu_AI1/1
  ground6/1 -> AO_trigger/1
  ground5/1 -> AI_trigger_3_4/1
  ground4/1 -> AI_trigger_1_2/1
  ground3/1 -> AO4/1
  ground2/1 -> AO3/1
  ground1/1 -> AO2/1
  ground/1 -> AO1/1
  dtc3/1 -> IO3xx PCI Write3/1
  sSpec3/1 -> dtc3/1
  cpu_AO4/1 -> sSpec3/1
  dtc2/1 -> IO3xx PCI Write2/1
  sSpec2/1 -> dtc2/1
  cpu_AO3/1 -> sSpec2/1
  dtc1/1 -> IO3xx PCI Write1/1
  sSpec1/1 -> dtc1/1
  cpu_AO2/1 -> sSpec1/1
  dtc/1 -> IO3xx PCI Write/1
  sSpec/1 -> dtc/1
  cpu_AO1/1 -> sSpec/1
  AI_valid_3_4/1 -> terminator5/1
  AI_valid_1_2/1 -> terminator4/1
  AI4/1 -> terminator3/1
  AI3/1 -> terminator2/1
  AI2/1 -> terminator1/1
  AI1/1 -> terminator/1

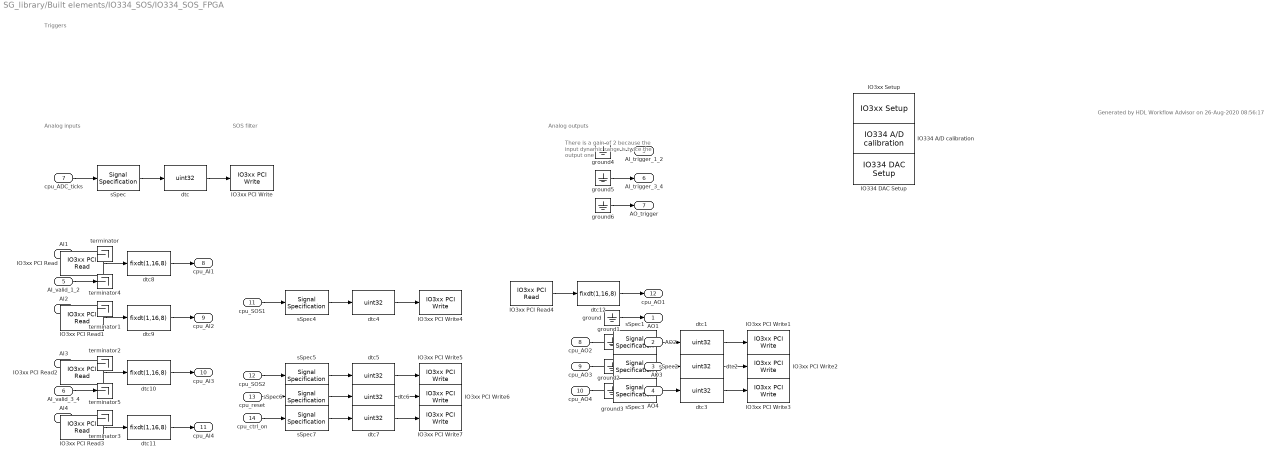
== system SG_library/Built elements/IO334_SOS/IO334_SOS_FPGA ==
  note: Generated by HDL Workflow Advisor on 26-Aug-2020 08:56:17
  note: There is a gain of 2 because the input dynamic range is twice the output one
  note: Analog inputs
  note: Triggers
  note: SOS filter
  note: Analog outputs
  AI1 : Inport
  AI2 : Inport  Port=2
  AI3 : Inport  Port=3
  AI4 : Inport  Port=4
  AI_valid_1_2 : Inport  Port=5
  AI_valid_3_4 : Inport  Port=6
  cpu_ADC_ticks : Inport  Port=7
  cpu_AO2 : Inport  Port=8
  cpu_AO3 : Inport  Port=9
  cpu_AO4 : Inport  Port=10
  cpu_SOS1 : Inport  Port=11
  cpu_SOS2 : Inport  Port=12
  cpu_reset : Inport  Port=13
  cpu_ctrl_on : Inport  Port=14
  IO334 A/D calibration : speedgoatlib_hdlCoder_IO3xx/IO334 A//D calibration  module_id=module_id
  IO334 DAC Setup : speedgoatlib_hdlCoder_IO3xx/IO334 DAC Setup  module_id=module_id  OutputRange=Auto (same as ADC)
  IO3xx PCI Read : speedgoatlib_hdlCoder_IO3xx/IO3xx PCI Read  device_id=deviceIdx  module_id=module_id  board_type=IO3xx  port_name=cpu_AI1  port_offset=hex2dec('118')  port_type=uint32  port_dim=1  strobe=0  sample_time=ts
  IO3xx PCI Read1 : speedgoatlib_hdlCoder_IO3xx/IO3xx PCI Read  device_id=deviceIdx  module_id=module_id  board_type=IO3xx  port_name=cpu_AI2  port_offset=hex2dec('11C')  port_type=uint32  port_dim=1  strobe=0  sample_time=ts
  IO3xx PCI Read2 : speedgoatlib_hdlCoder_IO3xx/IO3xx PCI Read  device_id=deviceIdx  module_id=module_id  board_type=IO3xx  port_name=cpu_AI3  port_offset=hex2dec('120')  port_type=uint32  port_dim=1  strobe=0  sample_time=ts
  IO3xx PCI Read3 : speedgoatlib_hdlCoder_IO3xx/IO3xx PCI Read  device_id=deviceIdx  module_id=module_id  board_type=IO3xx  port_name=cpu_AI4  port_offset=hex2dec('124')  port_type=uint32  port_dim=1  strobe=0  sample_time=ts
  IO3xx PCI Read4 : speedgoatlib_hdlCoder_IO3xx/IO3xx PCI Read  device_id=deviceIdx  module_id=module_id  board_type=IO3xx  port_name=cpu_AO1  port_offset=hex2dec('128')  port_type=uint32  port_dim=1  strobe=0  sample_time=ts
  IO3xx PCI Write : speedgoatlib_hdlCoder_IO3xx/IO3xx PCI Write  device_id=deviceIdx  module_id=module_id  board_type=IO3xx  port_name=cpu_ADC_ticks  port_offset=hex2dec('100')  port_type=uint32  port_dim=1  strobe=0  sample_time=ts
  IO3xx PCI Write1 : speedgoatlib_hdlCoder_IO3xx/IO3xx PCI Write  device_id=deviceIdx  module_id=module_id  board_type=IO3xx  port_name=cpu_AO2  port_offset=hex2dec('104')  port_type=uint32  port_dim=1  strobe=0  sample_time=ts
  IO3xx PCI Write2 : speedgoatlib_hdlCoder_IO3xx/IO3xx PCI Write  device_id=deviceIdx  module_id=module_id  board_type=IO3xx  port_name=cpu_AO3  port_offset=hex2dec('108')  port_type=uint32  port_dim=1  strobe=0  sample_time=ts
  IO3xx PCI Write3 : speedgoatlib_hdlCoder_IO3xx/IO3xx PCI Write  device_id=deviceIdx  module_id=module_id  board_type=IO3xx  port_name=cpu_AO4  port_offset=hex2dec('10C')  port_type=uint32  port_dim=1  strobe=0  sample_time=ts
  IO3xx PCI Write4 : speedgoatlib_hdlCoder_IO3xx/IO3xx PCI Write  device_id=deviceIdx  module_id=module_id  board_type=IO3xx  port_name=cpu_SOS1  port_offset=hex2dec('180')  port_type=uint32  port_dim=24  strobe=hex2dec('200')  sample_time=ts
  IO3xx PCI Write5 : speedgoatlib_hdlCoder_IO3xx/IO3xx PCI Write  device_id=deviceIdx  module_id=module_id  board_type=IO3xx  port_name=cpu_SOS2  port_offset=hex2dec('280')  port_type=uint32  port_dim=24  strobe=hex2dec('300')  sample_time=ts
  IO3xx PCI Write6 : speedgoatlib_hdlCoder_IO3xx/IO3xx PCI Write  device_id=deviceIdx  module_id=module_id  board_type=IO3xx  port_name=cpu_reset  port_offset=hex2dec('110')  port_type=uint32  port_dim=1  strobe=0  sample_time=ts
  IO3xx PCI Write7 : speedgoatlib_hdlCoder_IO3xx/IO3xx PCI Write  device_id=deviceIdx  module_id=module_id  board_type=IO3xx  port_name=cpu_ctrl_on  port_offset=hex2dec('114')  port_type=uint32  port_dim=1  strobe=0  sample_time=ts
  IO3xx Setup : speedgoatlib_hdlCoder_IO3xx/IO3xx Setup  mdl_ss_name=IO334_SOS_src/IO334_SOS/IO334_SOS_FPGA  board_type=IO334-325k  fpga_sync_mode=on  reset_mode=on  device_id=deviceIdx  module_id=module_id  pci_slot=slot  fpga_mat_file=C:\Speedgoat\Build\IO334_SOS\hdlsrc\IO334_SOS_src\IO334_SOS_FPGA.mat  timestamp_mcs=08/25/20 19:52:01  timestamp=2008251854  tsreg=hex2dec('8')  bsf_file=IO334_SOS_FPGA_2008251854.mcs  mcs=0
  dtc{,1..7} (8 alike) : DataTypeConversion  OutDataTypeStr=uint32  ConvertRealWorld=Stored Integer (SI)  RndMeth=Zero
  dtc{8..12} (5 alike) : DataTypeConversion  OutDataTypeStr=fixdt(1,16,8)  ConvertRealWorld=Stored Integer (SI)  RndMeth=Zero
  ground{,1..6} (7 alike) : Ground
  sSpec : SignalSpecification  OutDataTypeStr=fixdt(0,32,0)
  sSpec1 : SignalSpecification  OutDataTypeStr=fixdt(1,16,8)
  sSpec2 : SignalSpecification  OutDataTypeStr=fixdt(1,16,8)
  sSpec3 : SignalSpecification  OutDataTypeStr=fixdt(1,16,8)
  sSpec4 : SignalSpecification  OutDataTypeStr=fixdt(1,32,20)
  sSpec5 : SignalSpecification  OutDataTypeStr=fixdt(1,32,20)
  sSpec6 : SignalSpecification  OutDataTypeStr=fixdt('boolean')
  sSpec7 : SignalSpecification  OutDataTypeStr=fixdt('boolean')
  terminator{,1..5} (6 alike) : Terminator
  AO1 : Outport  VectorParamsAs1DForOutWhenUnconnected=off
  AO2 : Outport  Port=2  VectorParamsAs1DForOutWhenUnconnected=off
  AO3 : Outport  Port=3  VectorParamsAs1DForOutWhenUnconnected=off
  AO4 : Outport  Port=4  VectorParamsAs1DForOutWhenUnconnected=off
  AI_trigger_1_2 : Outport  Port=5  VectorParamsAs1DForOutWhenUnconnected=off
  AI_trigger_3_4 : Outport  Port=6  VectorParamsAs1DForOutWhenUnconnected=off
  AO_trigger : Outport  Port=7  VectorParamsAs1DForOutWhenUnconnected=off
  cpu_AI1 : Outport  Port=8  VectorParamsAs1DForOutWhenUnconnected=off
  cpu_AI2 : Outport  Port=9  VectorParamsAs1DForOutWhenUnconnected=off
  cpu_AI3 : Outport  Port=10  VectorParamsAs1DForOutWhenUnconnected=off
  cpu_AI4 : Outport  Port=11  VectorParamsAs1DForOutWhenUnconnected=off
  cpu_AO1 : Outport  Port=12  VectorParamsAs1DForOutWhenUnconnected=off
  wires:
  IO3xx PCI Read4/1 -> dtc12/1
  dtc12/1 -> cpu_AO1/1
  IO3xx PCI Read3/1 -> dtc11/1
  dtc11/1 -> cpu_AI4/1
  IO3xx PCI Read2/1 -> dtc10/1
  dtc10/1 -> cpu_AI3/1
  IO3xx PCI Read1/1 -> dtc9/1
  dtc9/1 -> cpu_AI2/1
  IO3xx PCI Read/1 -> dtc8/1
  dtc8/1 -> cpu_AI1/1
  ground6/1 -> AO_trigger/1
  ground5/1 -> AI_trigger_3_4/1
  ground4/1 -> AI_trigger_1_2/1
  ground3/1 -> AO4/1
  ground2/1 -> AO3/1
  ground1/1 -> AO2/1
  ground/1 -> AO1/1
  dtc7/1 -> IO3xx PCI Write7/1
  sSpec7/1 -> dtc7/1
  cpu_ctrl_on/1 -> sSpec7/1
  dtc6/1 -> IO3xx PCI Write6/1
  sSpec6/1 -> dtc6/1
  cpu_reset/1 -> sSpec6/1
  dtc5/1 -> IO3xx PCI Write5/1
  sSpec5/1 -> dtc5/1
  cpu_SOS2/1 -> sSpec5/1
  dtc4/1 -> IO3xx PCI Write4/1
  sSpec4/1 -> dtc4/1
  cpu_SOS1/1 -> sSpec4/1
  dtc3/1 -> IO3xx PCI Write3/1
  sSpec3/1 -> dtc3/1
  cpu_AO4/1 -> sSpec3/1
  dtc2/1 -> IO3xx PCI Write2/1
  sSpec2/1 -> dtc2/1
  cpu_AO3/1 -> sSpec2/1
  dtc1/1 -> IO3xx PCI Write1/1
  sSpec1/1 -> dtc1/1
  cpu_AO2/1 -> sSpec1/1
  dtc/1 -> IO3xx PCI Write/1
  sSpec/1 -> dtc/1
  cpu_ADC_ticks/1 -> sSpec/1
  AI_valid_3_4/1 -> terminator5/1
  AI_valid_1_2/1 -> terminator4/1
  AI4/1 -> terminator3/1
  AI3/1 -> terminator2/1
  AI2/1 -> terminator1/1
  AI1/1 -> terminator/1

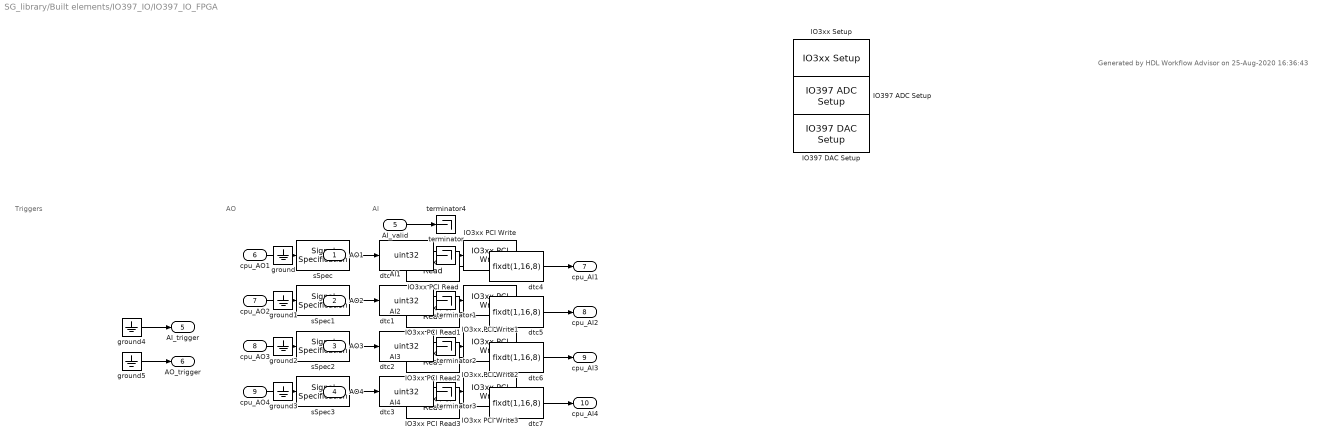
== system SG_library/Built elements/IO397_IO/IO397_IO_FPGA ==
  note: Generated by HDL Workflow Advisor on 25-Aug-2020 16:36:43
  note: Triggers
  note: AI
  note: AO
  AI1 : Inport
  AI2 : Inport  Port=2
  AI3 : Inport  Port=3
  AI4 : Inport  Port=4
  AI_valid : Inport  Port=5
  cpu_AO1 : Inport  Port=6
  cpu_AO2 : Inport  Port=7
  cpu_AO3 : Inport  Port=8
  cpu_AO4 : Inport  Port=9
  IO397 ADC Setup : speedgoatlib_hdlCoder_IO3xx/IO397 ADC Setup  module_id=module_id  range1=+-10 V  range2=+-10 V  range3=+-10 V  range4=+-10 V
  IO397 DAC Setup : speedgoatlib_hdlCoder_IO3xx/IO397 DAC Setup  module_id=module_id  span=+-10 V
  IO3xx PCI Read : speedgoatlib_hdlCoder_IO3xx/IO3xx PCI Read  device_id=deviceIdx  module_id=module_id  board_type=IO3xx  port_name=cpu_AI1  port_offset=hex2dec('110')  port_type=uint32  port_dim=1  strobe=0  sample_time=ts
  IO3xx PCI Read1 : speedgoatlib_hdlCoder_IO3xx/IO3xx PCI Read  device_id=deviceIdx  module_id=module_id  board_type=IO3xx  port_name=cpu_AI2  port_offset=hex2dec('114')  port_type=uint32  port_dim=1  strobe=0  sample_time=ts
  IO3xx PCI Read2 : speedgoatlib_hdlCoder_IO3xx/IO3xx PCI Read  device_id=deviceIdx  module_id=module_id  board_type=IO3xx  port_name=cpu_AI3  port_offset=hex2dec('118')  port_type=uint32  port_dim=1  strobe=0  sample_time=ts
  IO3xx PCI Read3 : speedgoatlib_hdlCoder_IO3xx/IO3xx PCI Read  device_id=deviceIdx  module_id=module_id  board_type=IO3xx  port_name=cpu_AI4  port_offset=hex2dec('11C')  port_type=uint32  port_dim=1  strobe=0  sample_time=ts
  IO3xx PCI Write : speedgoatlib_hdlCoder_IO3xx/IO3xx PCI Write  device_id=deviceIdx  module_id=module_id  board_type=IO3xx  port_name=cpu_AO1  port_offset=hex2dec('100')  port_type=uint32  port_dim=1  strobe=0  sample_time=ts
  IO3xx PCI Write1 : speedgoatlib_hdlCoder_IO3xx/IO3xx PCI Write  device_id=deviceIdx  module_id=module_id  board_type=IO3xx  port_name=cpu_AO2  port_offset=hex2dec('104')  port_type=uint32  port_dim=1  strobe=0  sample_time=ts
  IO3xx PCI Write2 : speedgoatlib_hdlCoder_IO3xx/IO3xx PCI Write  device_id=deviceIdx  module_id=module_id  board_type=IO3xx  port_name=cpu_AO3  port_offset=hex2dec('108')  port_type=uint32  port_dim=1  strobe=0  sample_time=ts
  IO3xx PCI Write3 : speedgoatlib_hdlCoder_IO3xx/IO3xx PCI Write  device_id=deviceIdx  module_id=module_id  board_type=IO3xx  port_name=cpu_AO4  port_offset=hex2dec('10C')  port_type=uint32  port_dim=1  strobe=0  sample_time=ts
  IO3xx Setup : speedgoatlib_hdlCoder_IO3xx/IO3xx Setup  mdl_ss_name=IO397_IO_src/IO397_IO/IO397_IO_FPGA  board_type=IO397-50k  fpga_sync_mode=on  reset_mode=on  device_id=deviceIdx  module_id=module_id  pci_slot=slot  fpga_mat_file=C:\Speedgoat\Build\IO397_IO\hdlsrc\IO397_IO_src\IO397_IO_FPGA.mat  timestamp_mcs=08/25/20 16:25:27  timestamp=2008251615  tsreg=hex2dec('8')  bsf_file=IO397_IO_FPGA_2008251615.mcs  mcs=0
  dtc{,1..3} (4 alike) : DataTypeConversion  OutDataTypeStr=uint32  ConvertRealWorld=Stored Integer (SI)  RndMeth=Zero
  dtc{4..7} (4 alike) : DataTypeConversion  OutDataTypeStr=fixdt(1,16,8)  ConvertRealWorld=Stored Integer (SI)  RndMeth=Zero
  ground{,1..5} (6 alike) : Ground
  sSpec{,1..3} (4 alike) : SignalSpecification  OutDataTypeStr=fixdt(1,16,8)
  terminator{,1..4} (5 alike) : Terminator
  AO1 : Outport  VectorParamsAs1DForOutWhenUnconnected=off
  AO2 : Outport  Port=2  VectorParamsAs1DForOutWhenUnconnected=off
  AO3 : Outport  Port=3  VectorParamsAs1DForOutWhenUnconnected=off
  AO4 : Outport  Port=4  VectorParamsAs1DForOutWhenUnconnected=off
  AI_trigger : Outport  Port=5  VectorParamsAs1DForOutWhenUnconnected=off
  AO_trigger : Outport  Port=6  VectorParamsAs1DForOutWhenUnconnected=off
  cpu_AI1 : Outport  Port=7  VectorParamsAs1DForOutWhenUnconnected=off
  cpu_AI2 : Outport  Port=8  VectorParamsAs1DForOutWhenUnconnected=off
  cpu_AI3 : Outport  Port=9  VectorParamsAs1DForOutWhenUnconnected=off
  cpu_AI4 : Outport  Port=10  VectorParamsAs1DForOutWhenUnconnected=off
  wires:
  IO3xx PCI Read3/1 -> dtc7/1
  dtc7/1 -> cpu_AI4/1
  IO3xx PCI Read2/1 -> dtc6/1
  dtc6/1 -> cpu_AI3/1
  IO3xx PCI Read1/1 -> dtc5/1
  dtc5/1 -> cpu_AI2/1
  IO3xx PCI Read/1 -> dtc4/1
  dtc4/1 -> cpu_AI1/1
  ground5/1 -> AO_trigger/1
  ground4/1 -> AI_trigger/1
  ground3/1 -> AO4/1
  ground2/1 -> AO3/1
  ground1/1 -> AO2/1
  ground/1 -> AO1/1
  dtc3/1 -> IO3xx PCI Write3/1
  sSpec3/1 -> dtc3/1
  cpu_AO4/1 -> sSpec3/1
  dtc2/1 -> IO3xx PCI Write2/1
  sSpec2/1 -> dtc2/1
  cpu_AO3/1 -> sSpec2/1
  dtc1/1 -> IO3xx PCI Write1/1
  sSpec1/1 -> dtc1/1
  cpu_AO2/1 -> sSpec1/1
  dtc/1 -> IO3xx PCI Write/1
  sSpec/1 -> dtc/1
  cpu_AO1/1 -> sSpec/1
  AI_valid/1 -> terminator4/1
  AI4/1 -> terminator3/1
  AI3/1 -> terminator2/1
  AI2/1 -> terminator1/1
  AI1/1 -> terminator/1
